simulink model "hcu_main_ADASwEPS"  (Simulink 8.2)
settings: Solver=FixedStepDiscrete  StartTime=0.0  StopTime=inf  FixedStep=0.001  RelTol=1e-3
PostLoadFcn:
  | , if any(exist('dsrtsu_mdlpostloadfcn', 'file') == [2, 3, 6]), try dsrtsu_mdlpostloadfcn('Execute', bdroot); catch fprintf('Error in PostLoadFcn (dsrtsu_mdlpostloadfcn) for model "%s":\n %s\n', bdroot, lasterr); end, end,
values from neighbouring files (symbols this model uses):
  C_TASK_1MS_S = (	C_TICK_TIME_S       )    [hcu_local_hdr.m]    (also in temp_ovrd_values.m = double(	0.001                  ))
  C_TASK_5MS_S = (	C_TICK_TIME_S      	)    [hcu_local_hdr.m]
  ENUM_ADASLFCSTATUS_OFF = uint8(  0  )    [hcu_local_hdr.m]
  ENUM_ADASLFCSTATUS_STANDBY = uint8(  1  )    [hcu_local_hdr.m]
  ENUM_ADASLKASTATUS_ACTIVE = uint8(  2  )    [hcu_local_hdr.m]
  ENUM_ADASLKASTATUS_OFF = uint8(  0  )    [hcu_local_hdr.m]
  ENUM_ADASLKASTATUS_STANDBY = uint8(  1  )    [hcu_local_hdr.m]
  ENUM_EPSMODEREQ_ANGLE = uint8(  1  )    [hcu_local_hdr.m]
  ENUM_EPSMODEREQ_INTERNAL = uint8(  0  )    [hcu_local_hdr.m]
  ENUM_EPSMODEREQ_TORQUE = uint8(  2  )    [hcu_local_hdr.m]
  ENUM_GEARPOSN_1ST = uint8(  1  )    [hcu_local_hdr.m]
  ENUM_GEARPOSN_2ND = uint8(  2  )    [hcu_local_hdr.m]
  ENUM_GEARPOSN_3RD = uint8(  3  )    [hcu_local_hdr.m]
  ENUM_GEARPOSN_4TH = uint8(  4  )    [hcu_local_hdr.m]
  ENUM_GEARPOSN_5TH = uint8(  5  )    [hcu_local_hdr.m]
  ENUM_GEARPOSN_6TH = uint8(  6  )    [hcu_local_hdr.m]
  ENUM_GEARPOSN_PN = uint8(  0  )    [hcu_local_hdr.m]
  ENUM_GEARPOSN_R = uint8(  7  )    [hcu_local_hdr.m]
  FALSE = boolean( 0 )    [hcu_local_hdr.m]
  TRUE = boolean( 1 )    [hcu_local_hdr.m]
undefined symbols (not defined in the file or in its folder): AACC_DistCtrlIMult_X_mps2, AACC_DistCtrlPMult_X_mps2, AACC_GearActual_enum, AACC_SpdCtrlIMult_X_mps2, AACC_SpdCtrlPMult_X_mps2, AACC_VehSpd_kph, AISP_EPSCurrent_pct, AISP_TqASensorDelta_pct, AISP_TqBSensorDelta_pct, ENUM_ACCSTATUS_ACTIVE, ENUM_ACCSTATUS_OFF, ENUM_ACCSTATUS_STANDBY, ENUM_ADASLFCSTATUS_ACTIVE, ENUM_ADASLFCSTATUS_TRANSITION, ENUM_LFCCCONTSTATUS_ACTIVE, ENUM_LFCCCONTSTATUS_NOTAVAIL_TEMP, ENUM_LFCCCONTSTATUS_OFF, ENUM_LFCCCONTSTATUS_READY, ENUM_LFCCCONTSTATUS_TRANSITION, ENUM_LKACCONTSTATUS_ACTIVE, ENUM_LKACCONTSTATUS_NOTAVAIL_TEMP, ENUM_LKACCONTSTATUS_OFF, ENUM_LKACCONTSTATUS_READY, KACC_AcclReqMax_g, KACC_AcclReqMin_g, KACC_ACCSetTimeGapDef1_s, KACC_ACCSetTimeGapDef2_s, KACC_ACCSetTimeGapDef3_s, KACC_ACCSetTimeGapDef4_s, KACC_ACCSetTimeGapDef5_s, KACC_AirDensity_kgpm3, KACC_AirDragCoef_rat, KACC_CommandsOn_flg, KACC_CruzSpdChgTimeThres_s, KACC_DecReqSwOffThres_Nm, KACC_DecReqSwOnThres_Nm, KACC_DistCtrlAdjTime_s, KACC_DistCtrlCalRate_s, KACC_DistCtrlIC_mps2, KACC_DistCtrlIGain_rat, KACC_DistCtrlIMax_mps2, KACC_DistCtrlIMin_mps2, KACC_DistCtrlIRest_flg, KACC_DistCtrlKGain_rat, KACC_DistCtrlPause_flg, KACC_DistCtrlPGain_rat, KACC_FinalDriveEff_pct, KACC_FinalDriveRatio_rat, KACC_FrontalArea_m2, KACC_GearBoxEff_pct, KACC_LongPushSpdChg_kph, KACC_MaxAccSetSpd_kph, KACC_MinAccSetSpd_kph, KACC_SetAllowSpdLim_kph, KACC_SpdCtrlAdjTime_s, KACC_SpdCtrlCalRate_s, KACC_SpdCtrlIC_mps2, KACC_SpdCtrlIGain_rat, KACC_SpdCtrlIMax_mps2, KACC_SpdCtrlIMin_mps2 ... (+26)
libraries: simulink x54, adas_lib x6, rti1401lib_dio_type3 x4, rtimmsu_dsrtlib x3, hcu_lib x2, aeb x1, ddm x1, dfr x1, dgi x1, dhp x1, dinr x1, dip x1
(part 9 of 9)

== system hcu_main_ADASwEPS/APPH/ACC/ACC/ACCStrategy/Torque Estimation/TqConverter ==
  TqIn_TC : Inport
  OmegaIn_TC : Inport  Port=2
  VDINR_EngSpd_rpm : Inport  Port=3
  Gain : Gain  Gain=2*pi/60
  Product1 : Product  Inputs=**  RndMeth=Zero
  Product3 : Product  Inputs=*/  RndMeth=Zero
  TorqueRatio : Lookup  InputValues=[0 0.1 0.202 0.301 0.402 0.503 0.621 0.654 0.702 0.751 0.8 0.821 0.842 0.861 0.882 0.901 0.921]  Table=|  LookUpMeth=Interpolation-Use End Values
      | [1.88 1.81 1.73 1.64 1.53 1.41 1.28 1.25 1.2 1.15 1.1 1.08 1.06 1.04 1.01 1 1
      | ]
  VACC_TqReqRaw_Nm : Outport
  wires:
  Product1/1 -> VACC_TqReqRaw_Nm/1  "VACC_TqReqRaw_Nm"
  VDINR_EngSpd_rpm/1 -> Gain/1
  OmegaIn_TC/1 -> Product3/1
  Product3/1 -> TorqueRatio/1
  TorqueRatio/1 -> Product1/2
  TqIn_TC/1 -> Product1/1
  Gain/1 -> Product3/2

== system hcu_main_ADASwEPS/APPH/ACC/ACC/ACCStrategy/Trigger signal generator/trigger signal generator ==
  Time_dur [s] : Inport
  Constant3 : Constant  Value=0  OutDataTypeStr=single
  Constant4 : Constant  Value=C_TASK_5MS_S
  Relational Operator1 : RelationalOperator  OutDataTypeStr=boolean
  Sum1 : Sum  Inputs=|++  SaturateOnIntegerOverflow=on  InputSameDT=on
  Sum2 : Sum  Inputs=+-
  Switch3 : Switch  Threshold=0.5
  Unit Delay2 : UnitDelay  SampleTime=-1
  Unit Delay3 : UnitDelay  SampleTime=-1
  Trigger_signal : Outport  OutputWhenDisabled=reset  InitialOutput=[0]
  wires:
  Sum2/1 -> Relational Operator1/2
  Unit Delay3/1 -> Switch3/2
  Unit Delay2/1 -> Sum1/2
  Switch3/1 -> Relational Operator1/1, Unit Delay2/1
  Constant3/1 -> Switch3/1
  Time_dur [s]/1 -> Sum2/1
  Relational Operator1/1 -> Unit Delay3/1, Trigger_signal/1
  Constant4/1 -> Sum2/2, Sum1/1
  Sum1/1 -> Switch3/3

== system hcu_main_ADASwEPS/APPH/ACC/ACC/ACCStrategy/Vehicle Acceleration Calculation/signal_filter ==
  raw_input : Inport
  Tc : Inport  Port=2
  Ts : Inport  Port=3
  FirstOrderFilter : Subsystem  RTWFileName=HCU_LIB
      settings: RTWFileNameOpts=User specified
  IC : UnitDelay  Tag=struct('comment',struct('text','','placement',1),'logdata',struct('maxnumvals',inf,'plotchannels',[],'stepsize',0,'downsampling',1,'loggingmode',3,'channels',1),'output',struct('width',1,'name','$S_$B','unit','','type','Int16','offset',0,'max',NaN,'min',NaN,'freeze',1,'lsb',1,'arb',0,'class','default','address','','description','','autoscalingmode',1,'lowerheadroom',1,'upperheadroom',1,'headroomunit','bit','checkmin',0,'checkmax',0,'show',0,'initial','2'),'state',0,'dt','-1','date',731455.586925799)  SampleTime=-1
  Switch1 : Switch  Tag=struct('comment',struct('text','','placement',1),'logdata',struct('maxnumvals',inf,'plotchannels',[],'stepsize',0,'downsampling',1,'loggingmode',3,'channels',1),'output',struct('width',1,'name','$S_$B','unit','','type','Int32Bin15','offset',0,'max',65535,'min',-65536,'freeze',1,'lsb',2^-15,'arb',0,'class','default','address','','description','','autoscalingmode',1,'lowerheadroom',1,'upperheadroom',1,'headroomunit','bit','checkmin',0,'checkmax',0,'show',0),'threshold',struct('width',1,'name','$S_$B_threshold','unit','','type','Int16','offset',0,'max',NaN,'min',NaN,'freeze',1,'lsb',1,'arb',0,'class','default','address','','description','','value','1','scalar',0),'date',731455.58657044)  Threshold=0.5  InputSameDT=on
  zero : Constant  Tag=struct('comment',struct('text','','placement',1),'output',struct('width',1,'name','$S_$B','unit','','type','Int16','offset',0,'max',NaN,'min',NaN,'freeze',1,'lsb',1,'arb',0,'class','default','address','','description','','value','0','tolerance',1,'show',0),'date',731455.58675544)  Value=TRUE
  zero1 : Constant  Tag=struct('comment',struct('text','','placement',1),'output',struct('width',1,'name','$S_$B','unit','','type','Int16','offset',0,'max',NaN,'min',NaN,'freeze',1,'lsb',1,'arb',0,'class','default','address','','description','','value','0','tolerance',1,'show',0),'date',731455.58675544)  Value=0  OutDataTypeStr=single
  raw_input_filt : Outport
  wires:
  zero/1 -> IC/1
  raw_input/1 -> FirstOrderFilter/1(in)
  Tc/1 -> Switch1/1
  Ts/1 -> FirstOrderFilter/3(Ts)
  IC/1 -> Switch1/2
  FirstOrderFilter/1(out) -> raw_input_filt/1
  Switch1/1 -> FirstOrderFilter/2(Tc)
  zero1/1 -> Switch1/3

== system hcu_main_ADASwEPS/EPSS/EPSS/AngleMode/Angle2Torque/Rate_Limit/RateLimiter ==
  Data_Input : Inport
  Rising Rate : Inport  Port=2
  Falling Rate : Inport  Port=3
  Initial_Condition : Inport  Port=4
  Chart : Stateflow chart  TreatAsAtomicUnit=on
  Constant : Constant  Value=C_TASK_1MS_S
  Constant1 : Constant  Value=C_TASK_1MS_S
  Constant4 : Constant
  Constant5 : Constant
  Data Type Conversion : DataTypeConversion  OutDataTypeStr=boolean
  Data Type Conversion1 : DataTypeConversion  OutDataTypeStr=boolean
  Product{1..4} (4 alike) : Product  Inputs=*/  RndMeth=Zero
  Relational Operator : RelationalOperator  Operator=>  OutDataTypeStr=boolean
  Relational Operator1 : RelationalOperator  Operator=<  OutDataTypeStr=boolean
  Saturation : Subsystem
  Sum1 : Sum  Inputs=|++
  Switch1 : Switch  Threshold=0.5
  Unit Delay1 : UnitDelay  SampleTime=-1
  Data_Output : Outport
  wires:
  Relational Operator1/1 -> Data Type Conversion/1
  Relational Operator/1 -> Data Type Conversion1/1
  Data_Input/1 -> Relational Operator/1, Relational Operator1/1, Chart/3(Data_in)
  Product3/1 -> Product1/2
  Product4/1 -> Product2/2
  Product1/1 -> Chart/4(increase_tou)
  Product2/1 -> Chart/5(decrease_tou)
  Data Type Conversion/1 -> Chart/2(decrease)
  Data Type Conversion1/1 -> Chart/1(increase)
  Chart/2(tou) -> Sum1/1
  Saturation/1(out) -> Switch1/3
  Chart/3(Min) -> Saturation/2(min)
  Chart/4(Max) -> Saturation/3(max)
  Chart/1(Initial) -> Switch1/2
  Initial_Condition/1 -> Switch1/1
  Constant/1 -> Product3/2
  Constant4/1 -> Product3/1
  Constant1/1 -> Product4/2
  Constant5/1 -> Product4/1
  Switch1/1 -> Data_Output/1, Unit Delay1/1
  Rising Rate/1 -> Product1/1
  Falling Rate/1 -> Product2/1
  Sum1/1 -> Saturation/1(in)
  Unit Delay1/1 -> Sum1/2, Relational Operator/2, Relational Operator1/2

== system hcu_main_ADASwEPS/APPH/ACC/ACC/ACCStrategy/Distance Control/PI Controller for Distance Control/Integrator ==
  In : Inport
  Rst : Inport  Port=2
  IC : Inport  Port=3
  Min : Inport  Port=4
  Max : Inport  Port=5
  Constant : Constant  Value=C_TASK_5MS_S  OutDataTypeStr=single
  Data Type Conversion : DataTypeConversion  OutDataTypeStr=boolean  RndMeth=Zero
  Product : Product  SaturateOnIntegerOverflow=on  InputSameDT=on  OutDataTypeStr=Inherit: Same as first input
  Saturation : Subsystem
  Sum : Sum  Inputs=++|  SaturateOnIntegerOverflow=on  InputSameDT=on
  Switch1 : Switch  Threshold=1  ZeroCross=off  SaturateOnIntegerOverflow=on  InputSameDT=on
  Unit Delay : UnitDelay  SampleTime=-1
  Out : Outport
  wires:
  IC/1 -> Switch1/1
  Max/1 -> Saturation/3(max)
  Min/1 -> Saturation/2(min)
  Data Type Conversion/1 -> Switch1/2
  Rst/1 -> Data Type Conversion/1
  Unit Delay/1 -> Switch1/3
  Product/1 -> Sum/2
  In/1 -> Product/1
  Constant/1 -> Product/2
  Switch1/1 -> Sum/1, Out/1
  Sum/1 -> Saturation/1(in)
  Saturation/1(out) -> Unit Delay/1

== system hcu_main_ADASwEPS/APPH/ACC/ACC/ACCStrategy/Distance Control/Trigger signal generator/trigger signal generator ==
  Time_dur [s] : Inport
  Constant3 : Constant  Value=0  OutDataTypeStr=single
  Constant4 : Constant  Value=C_TASK_5MS_S
  Relational Operator1 : RelationalOperator  OutDataTypeStr=boolean
  Sum1 : Sum  Inputs=|++  SaturateOnIntegerOverflow=on  InputSameDT=on
  Sum2 : Sum  Inputs=+-
  Switch3 : Switch  Threshold=0.5
  Unit Delay2 : UnitDelay  SampleTime=-1
  Unit Delay3 : UnitDelay  SampleTime=-1
  Trigger_signal : Outport  OutputWhenDisabled=reset  InitialOutput=[0]
  wires:
  Sum2/1 -> Relational Operator1/2
  Unit Delay3/1 -> Switch3/2
  Unit Delay2/1 -> Sum1/2
  Switch3/1 -> Relational Operator1/1, Unit Delay2/1
  Constant3/1 -> Switch3/1
  Time_dur [s]/1 -> Sum2/1
  Relational Operator1/1 -> Unit Delay3/1, Trigger_signal/1
  Constant4/1 -> Sum2/2, Sum1/1
  Sum1/1 -> Switch3/3

== system hcu_main_ADASwEPS/APPH/ACC/ACC/ACCStrategy/Distance Control/Trigger signal generator1/trigger signal generator ==
  Time_dur [s] : Inport
  Constant3 : Constant  Value=0  OutDataTypeStr=single
  Constant4 : Constant  Value=C_TASK_5MS_S
  Relational Operator1 : RelationalOperator  OutDataTypeStr=boolean
  Sum1 : Sum  Inputs=|++  SaturateOnIntegerOverflow=on  InputSameDT=on
  Sum2 : Sum  Inputs=+-
  Switch3 : Switch  Threshold=0.5
  Unit Delay2 : UnitDelay  SampleTime=-1
  Unit Delay3 : UnitDelay  SampleTime=-1
  Trigger_signal : Outport  OutputWhenDisabled=reset  InitialOutput=[0]
  wires:
  Sum2/1 -> Relational Operator1/2
  Unit Delay3/1 -> Switch3/2
  Unit Delay2/1 -> Sum1/2
  Switch3/1 -> Relational Operator1/1, Unit Delay2/1
  Constant3/1 -> Switch3/1
  Time_dur [s]/1 -> Sum2/1
  Relational Operator1/1 -> Unit Delay3/1, Trigger_signal/1
  Constant4/1 -> Sum2/2, Sum1/1
  Sum1/1 -> Switch3/3

== system hcu_main_ADASwEPS/APPH/ACC/ACC/ACCStrategy/Distance Control/Vehicle Acceleration Calculation/signal_filter ==
  raw_input : Inport
  Tc : Inport  Port=2
  Ts : Inport  Port=3
  FirstOrderFilter : Subsystem  RTWFileName=HCU_LIB
      settings: RTWFileNameOpts=User specified
  IC : UnitDelay  Tag=struct('comment',struct('text','','placement',1),'logdata',struct('maxnumvals',inf,'plotchannels',[],'stepsize',0,'downsampling',1,'loggingmode',3,'channels',1),'output',struct('width',1,'name','$S_$B','unit','','type','Int16','offset',0,'max',NaN,'min',NaN,'freeze',1,'lsb',1,'arb',0,'class','default','address','','description','','autoscalingmode',1,'lowerheadroom',1,'upperheadroom',1,'headroomunit','bit','checkmin',0,'checkmax',0,'show',0,'initial','2'),'state',0,'dt','-1','date',731455.586925799)  SampleTime=-1
  Switch1 : Switch  Tag=struct('comment',struct('text','','placement',1),'logdata',struct('maxnumvals',inf,'plotchannels',[],'stepsize',0,'downsampling',1,'loggingmode',3,'channels',1),'output',struct('width',1,'name','$S_$B','unit','','type','Int32Bin15','offset',0,'max',65535,'min',-65536,'freeze',1,'lsb',2^-15,'arb',0,'class','default','address','','description','','autoscalingmode',1,'lowerheadroom',1,'upperheadroom',1,'headroomunit','bit','checkmin',0,'checkmax',0,'show',0),'threshold',struct('width',1,'name','$S_$B_threshold','unit','','type','Int16','offset',0,'max',NaN,'min',NaN,'freeze',1,'lsb',1,'arb',0,'class','default','address','','description','','value','1','scalar',0),'date',731455.58657044)  Threshold=0.5  InputSameDT=on
  zero : Constant  Tag=struct('comment',struct('text','','placement',1),'output',struct('width',1,'name','$S_$B','unit','','type','Int16','offset',0,'max',NaN,'min',NaN,'freeze',1,'lsb',1,'arb',0,'class','default','address','','description','','value','0','tolerance',1,'show',0),'date',731455.58675544)  Value=TRUE
  zero1 : Constant  Tag=struct('comment',struct('text','','placement',1),'output',struct('width',1,'name','$S_$B','unit','','type','Int16','offset',0,'max',NaN,'min',NaN,'freeze',1,'lsb',1,'arb',0,'class','default','address','','description','','value','0','tolerance',1,'show',0),'date',731455.58675544)  Value=0  OutDataTypeStr=single
  raw_input_filt : Outport
  wires:
  zero/1 -> IC/1
  raw_input/1 -> FirstOrderFilter/1(in)
  Tc/1 -> Switch1/1
  Ts/1 -> FirstOrderFilter/3(Ts)
  IC/1 -> Switch1/2
  FirstOrderFilter/1(out) -> raw_input_filt/1
  Switch1/1 -> FirstOrderFilter/2(Tc)
  zero1/1 -> Switch1/3

== system hcu_main_ADASwEPS/APPH/ACC/ACC/ACCStrategy/Speed Control/PI Controller for Seepd Control/Integrator ==
  In : Inport
  Rst : Inport  Port=2
  IC : Inport  Port=3
  Min : Inport  Port=4
  Max : Inport  Port=5
  Constant : Constant  Value=C_TASK_5MS_S  OutDataTypeStr=single
  Data Type Conversion : DataTypeConversion  OutDataTypeStr=boolean  RndMeth=Zero
  Product : Product  SaturateOnIntegerOverflow=on  InputSameDT=on  OutDataTypeStr=Inherit: Same as first input
  Saturation : Subsystem
  Sum : Sum  Inputs=++|  SaturateOnIntegerOverflow=on  InputSameDT=on
  Switch1 : Switch  Threshold=1  ZeroCross=off  SaturateOnIntegerOverflow=on  InputSameDT=on
  Unit Delay : UnitDelay  SampleTime=-1
  Out : Outport
  wires:
  IC/1 -> Switch1/1
  Max/1 -> Saturation/3(max)
  Min/1 -> Saturation/2(min)
  Data Type Conversion/1 -> Switch1/2
  Rst/1 -> Data Type Conversion/1
  Unit Delay/1 -> Switch1/3
  Product/1 -> Sum/2
  In/1 -> Product/1
  Constant/1 -> Product/2
  Switch1/1 -> Sum/1, Out/1
  Sum/1 -> Saturation/1(in)
  Saturation/1(out) -> Unit Delay/1

== system hcu_main_ADASwEPS/APPH/ACC/ACC/ACCStrategy/Speed Control/Trigger signal generator/trigger signal generator ==
  Time_dur [s] : Inport
  Constant3 : Constant  Value=0  OutDataTypeStr=single
  Constant4 : Constant  Value=C_TASK_5MS_S
  Relational Operator1 : RelationalOperator  OutDataTypeStr=boolean
  Sum1 : Sum  Inputs=|++  SaturateOnIntegerOverflow=on  InputSameDT=on
  Sum2 : Sum  Inputs=+-
  Switch3 : Switch  Threshold=0.5
  Unit Delay2 : UnitDelay  SampleTime=-1
  Unit Delay3 : UnitDelay  SampleTime=-1
  Trigger_signal : Outport  OutputWhenDisabled=reset  InitialOutput=[0]
  wires:
  Sum2/1 -> Relational Operator1/2
  Unit Delay3/1 -> Switch3/2
  Unit Delay2/1 -> Sum1/2
  Switch3/1 -> Relational Operator1/1, Unit Delay2/1
  Constant3/1 -> Switch3/1
  Time_dur [s]/1 -> Sum2/1
  Relational Operator1/1 -> Unit Delay3/1, Trigger_signal/1
  Constant4/1 -> Sum2/2, Sum1/1
  Sum1/1 -> Switch3/3

== system hcu_main_ADASwEPS/APPH/ACC/ACC/ACCStrategy/Torque Estimation/Tire/Derivative ==
  SampleTime : Inport
  Omega_tire : Inport  Port=2
  Trigger : TriggerPort
  Divide : Product  Inputs=*/
  Mux1 : Mux  Inputs=2
  Scope1 : Scope
      settings: SaveName=ScopeData9
  Subtract : Sum  Inputs=+-
  Unit Delay : UnitDelay  SampleTime=-1
  AlphaOut_tire : Outport
  wires:
  Omega_tire/1 -> Subtract/1, Unit Delay/1
  Divide/1 -> AlphaOut_tire/1
  SampleTime/1 -> Divide/2
  Subtract/1 -> Divide/1, Mux1/1
  Unit Delay/1 -> Subtract/2, Mux1/2
  Mux1/1 -> Scope1/1

== system hcu_main_ADASwEPS/APPH/ACC/ACC/ACCStrategy/Torque Estimation/Tire/trigger signal generator ==
  Time_dur [s] : Inport
  Constant3 : Constant  Value=single(0)
  Constant4 : Constant  Value=C_TASK_5MS_S
  Relational Operator1 : RelationalOperator  OutDataTypeStr=boolean
  Sum1 : Sum  Inputs=|++  SaturateOnIntegerOverflow=on  InputSameDT=on
  Sum2 : Sum  Inputs=+-
  Switch3 : Switch  Threshold=0.5
  Unit Delay2 : UnitDelay  InitialCondition=single(0)  SampleTime=-1
  Unit Delay3 : UnitDelay  SampleTime=-1
  Trigger_signal : Outport  OutputWhenDisabled=reset  InitialOutput=[0]
  wires:
  Sum1/1 -> Switch3/3
  Constant4/1 -> Sum1/1, Sum2/2
  Relational Operator1/1 -> Trigger_signal/1, Unit Delay3/1
  Time_dur [s]/1 -> Sum2/1
  Constant3/1 -> Switch3/1
  Switch3/1 -> Unit Delay2/1, Relational Operator1/1
  Unit Delay2/1 -> Sum1/2
  Unit Delay3/1 -> Switch3/2
  Sum2/1 -> Relational Operator1/2

== system hcu_main_ADASwEPS/APPH/ACC/ACC/ACCStrategy/Vehicle Acceleration Calculation/signal_filter/FirstOrderFilter ==
  in : Inport
  Tc : Inport  Port=2
  Ts : Inport  Port=3
  Add : Sum
  Add1 : Sum
  Add2 : Sum  Inputs=+-
  Constant : Constant  OutDataTypeStr=single
  Divide : Product  Inputs=*/
  Product : Product  RndMeth=Zero
  Product1 : Product  RndMeth=Zero
  Unit Delay : UnitDelay  SampleTime=-1
  out : Outport
  wires:
  Add/1 -> Unit Delay/1, out/1
  Product1/1 -> Add/2
  Product/1 -> Add/1
  Add2/1 -> Product/2
  in/1 -> Product/1
  Divide/1 -> Product1/1, Add2/2
  Constant/1 -> Add2/1
  Add1/1 -> Divide/2
  Ts/1 -> Add1/2
  Tc/1 -> Divide/1, Add1/1
  Unit Delay/1 -> Product1/2

== system hcu_main_ADASwEPS/EPSS/EPSS/AngleMode/Angle2Torque/Rate_Limit/RateLimiter/Saturation ==
  in : Inport
  min : Inport  Port=2
  max : Inport  Port=3
  MinMax : MinMax  Function=max  Inputs=2  ZeroCross=off  SaturateOnIntegerOverflow=on  InputSameDT=on
  MinMax1 : MinMax  Inputs=2  ZeroCross=off  SaturateOnIntegerOverflow=on  InputSameDT=on
  out : Outport
  wires:
  MinMax1/1 -> out/1
  max/1 -> MinMax1/2
  min/1 -> MinMax/2
  in/1 -> MinMax/1
  MinMax/1 -> MinMax1/1

== system hcu_main_ADASwEPS/APPH/ACC/ACC/ACCStrategy/Distance Control/PI Controller for Distance Control/Integrator/Saturation ==
  in : Inport
  min : Inport  Port=2
  max : Inport  Port=3
  MinMax : MinMax  Function=max  Inputs=2  ZeroCross=off  SaturateOnIntegerOverflow=on  InputSameDT=on
  MinMax1 : MinMax  Inputs=2  ZeroCross=off  SaturateOnIntegerOverflow=on  InputSameDT=on
  out : Outport
  wires:
  MinMax/1 -> MinMax1/1
  in/1 -> MinMax/1
  min/1 -> MinMax/2
  max/1 -> MinMax1/2
  MinMax1/1 -> out/1

== system hcu_main_ADASwEPS/APPH/ACC/ACC/ACCStrategy/Distance Control/Vehicle Acceleration Calculation/signal_filter/FirstOrderFilter ==
  in : Inport
  Tc : Inport  Port=2
  Ts : Inport  Port=3
  Add : Sum
  Add1 : Sum
  Add2 : Sum  Inputs=+-
  Constant : Constant  OutDataTypeStr=single
  Divide : Product  Inputs=*/
  Product : Product  RndMeth=Zero
  Product1 : Product  RndMeth=Zero
  Unit Delay : UnitDelay  SampleTime=-1
  out : Outport
  wires:
  Add/1 -> Unit Delay/1, out/1
  Product1/1 -> Add/2
  Product/1 -> Add/1
  Add2/1 -> Product/2
  in/1 -> Product/1
  Divide/1 -> Product1/1, Add2/2
  Constant/1 -> Add2/1
  Add1/1 -> Divide/2
  Ts/1 -> Add1/2
  Tc/1 -> Divide/1, Add1/1
  Unit Delay/1 -> Product1/2

== system hcu_main_ADASwEPS/APPH/ACC/ACC/ACCStrategy/Speed Control/PI Controller for Seepd Control/Integrator/Saturation ==
  in : Inport
  min : Inport  Port=2
  max : Inport  Port=3
  MinMax : MinMax  Function=max  Inputs=2  ZeroCross=off  SaturateOnIntegerOverflow=on  InputSameDT=on
  MinMax1 : MinMax  Inputs=2  ZeroCross=off  SaturateOnIntegerOverflow=on  InputSameDT=on
  out : Outport
  wires:
  MinMax/1 -> MinMax1/1
  in/1 -> MinMax/1
  min/1 -> MinMax/2
  max/1 -> MinMax1/2
  MinMax1/1 -> out/1

== stateflow chart APPH/Scheduler ==
  (default) -> (junction 23)
  (junction 23) -> (junction 24) : {
      | trig_PMM; ...
      | trig_DGI; ...
      | trig_DINR; ...
      | trig_TRCK; ...
      | trig_DDM; ...
      | trig_DHP; ...
      | trig_EID; ...
      | trig_LANE; ...
      | trig_SFTY; ...
      | trig_FST; ...
      | trig_LFCM; ...
      | trig_STR; ...
      | trig_OBJ; ...
      | trig_PTH; ...
      | trig_MCT;...
      | trig_TTC; ...
      | trig_AEB; ...
      | trig_ACC; ...
      | trig_DIP; ...
      | trig_DFR; ...
      | }
  events: trig_PMM output FUNCTION_CALL_EVENT; trig_DGI output FUNCTION_CALL_EVENT; trig_DINR output FUNCTION_CALL_EVENT; trig_TRCK output FUNCTION_CALL_EVENT; trig_DDM output FUNCTION_CALL_EVENT; trig_DHP output FUNCTION_CALL_EVENT; trig_EID output FUNCTION_CALL_EVENT; trig_LANE output FUNCTION_CALL_EVENT; trig_SFTY output FUNCTION_CALL_EVENT; trig_FST output FUNCTION_CALL_EVENT; trig_LFCM output FUNCTION_CALL_EVENT; trig_STR output FUNCTION_CALL_EVENT; trig_OBJ output FUNCTION_CALL_EVENT; trig_PTH output FUNCTION_CALL_EVENT; trig_MCT output FUNCTION_CALL_EVENT; trig_TTC output FUNCTION_CALL_EVENT; trig_AEB output FUNCTION_CALL_EVENT; trig_ACC output FUNCTION_CALL_EVENT; trig_DIP output FUNCTION_CALL_EVENT; trig_DFR output FUNCTION_CALL_EVENT

== stateflow chart APPH/ACC/ACC/ACCStatus_SetSpeed_SetTimeGap/ACC_SetSpeed_Determination ==
  state ACCOff
    en:VACC_ACCSetSpd_kph=0;
    en:VACC_ACCSetSpdIni_kph=0;
    en:CurrSetSpd=0;
  state Initialize
    en:VACC_ACCSetSpd_kph=0;
    en:VACC_ACCSetSpdIni_kph=0;
    en:CurrSetSpd=0;
  state ACCOn
    state SetOn
      en:VACC_ACCSetSpd_kph=VDINR_VehSpd_kph;
      en:VACC_ACCSetSpdIni_kph=VDINR_VehSpd_kph;
      en:CurrSetSpd=VDINR_VehSpd_kph;
    state SetOn_HighSpeed
      en:VACC_ACCSetSpd_kph=VACC_MaxAccSetSpd_kph;
      en:VACC_ACCSetSpdIni_kph=VACC_MaxAccSetSpd_kph;
      en:CurrSetSpd=VACC_MaxAccSetSpd_kph;
    state SetOn_LowSpeed
      en:VACC_ACCSetSpd_kph=VACC_MinAccSetSpd_kph;
      en:VACC_ACCSetSpdIni_kph=VACC_MinAccSetSpd_kph;
      en:CurrSetSpd=VACC_MinAccSetSpd_kph;
    state ResOn
      en:VACC_ACCSetSpd_kph=VACC_ACCSetSpdLast_kph;
      en:VACC_ACCSetSpdIni_kph=VACC_ACCSetSpdLast_kph;
      en:CurrSetSpd=VACC_ACCSetSpdLast_kph;
    state WaitforACCActive
      en:VACC_ACCSetSpd_kph=CurrSetSpd;
      en:VACC_ACCSetSpdIni_kph=CurrSetSpd;
    state BrakeSet_LowSpeed
      en:VACC_ACCSetSpd_kph=VACC_MinAccSetSpd_kph;
      en:VACC_ACCSetSpdIni_kph=VACC_MinAccSetSpd_kph;
      en:CurrSetSpd=VACC_MinAccSetSpd_kph;
    state BrakeSet_NormalSpeed
      en:VACC_ACCSetSpd_kph=CurrSetSpd;
      en:VACC_ACCSetSpdIni_kph=CurrSetSpd;
    state SpeedSet
      state WaitingForSpdChange
        en:VACC_ACCSetSpd_kph=CurrSetSpd;
        en:VACC_ACCSetSpdIni_kph=CurrSetSpd;
      state PrepareToDec
      state PrepareToInc
      state DecreaseToMin
        en: CurrSetSpd=VACC_MinAccSetSpd_kph;
        en: VACC_ACCSetSpd_kph=CurrSetSpd;
      state Decrease1
        ex: CurrSetSpd=CurrSetSpd-1;
      state Decrease11
        en: CurrSetSpd=CurrSetSpd-VACC_LongPushSpdChg_kph;
        en: VACC_ACCSetSpd_kph=CurrSetSpd;
      state Increase1
        ex: CurrSetSpd=CurrSetSpd+1;
      state SetSpeedUpLimit
        ex: CurrSetSpd=VOBU_SetSpdUplim_kph;
      (default) -> WaitingForSpdChange
      SetSpeedUpLimit -> WaitingForSpdChange
      Increase1 -> WaitingForSpdChange
      (junction 89) -> WaitingForSpdChange [order 2]
      WaitingForSpdChange -> PrepareToInc [order 2] : [VACC_ACCResSpdIncVCU_flg]
      (junction 90) -> WaitingForSpdChange [order 2]
      DecreaseToMin -> WaitingForSpdChange : [!VACC_ACCSetSpdDecVCU_flg]
      Decrease11 -> WaitingForSpdChange [order 2] : [!VACC_ACCSetSpdDecVCU_flg]
      WaitingForSpdChange -> PrepareToDec [order 1] : [VACC_ACCSetSpdDecVCU_flg]
      (junction 88) -> WaitingForSpdChange [order 2]
      Decrease1 -> WaitingForSpdChange
      PrepareToDec -> (junction 86) [order 2] : after(VACC_CruzSpdChgTimeThres_s/C_TASK_5MS_S,tick) ...
          | [VACC_ACCSetSpdDecVCU_flg]
      (junction 86) -> (junction 87) [order 1] : [CurrSetSpd>=(VACC_MinAccSetSpd_kph+1) && ...
          |  CurrSetSpd<(VACC_MinAccSetSpd_kph+VACC_LongPushSpdChg_kph)]
      PrepareToInc -> (junction 90) [order 1] : after(VACC_CruzSpdChgTimeThres_s/C_TASK_5MS_S,tick)...
          | [!VACC_ACCResSpdIncVCU_flg]
      (junction 86) -> Decrease11 [order 2] : [CurrSetSpd>=(VACC_MinAccSetSpd_kph+VACC_LongPushSpdChg_kph)]
      (junction 87) -> DecreaseToMin
      PrepareToDec -> (junction 88) [order 1] : [!VACC_ACCSetSpdDecVCU_flg]
      PrepareToInc -> (junction 89) [order 2] : [!VACC_ACCResSpdIncVCU_flg]
      (junction 88) -> Decrease1 [order 1] : [CurrSetSpd>=(VACC_MinAccSetSpd_kph+1)]
      (junction 89) -> Increase1 [order 1] : [CurrSetSpd<=(VACC_MaxAccSetSpd_kph-1)]
      (junction 93) -> Decrease11
      (junction 90) -> (junction 94) [order 1] : [CurrSetSpd<=(VOBU_SetSpdUplim_kph)]
      Decrease11 -> (junction 92) [order 1] : after(VACC_CruzSpdChgTimeThres_s/C_TASK_5MS_S,tick) ...
          | [VACC_ACCSetSpdDecVCU_flg]
      (junction 91) -> DecreaseToMin
      (junction 92) -> (junction 91) [order 1] : [CurrSetSpd>=(VACC_MinAccSetSpd_kph+1) && ...
          |  CurrSetSpd<(VACC_MinAccSetSpd_kph+VACC_LongPushSpdChg_kph)]
      (junction 92) -> (junction 93) [order 2] : [CurrSetSpd>=(VACC_MinAccSetSpd_kph+VACC_LongPushSpdChg_kph)]
      (junction 94) -> SetSpeedUpLimit
    (default) -> WaitforACCActive
    (junction 48) -> WaitforACCActive
    (junction 59) -> (junction 48)
    WaitforACCActive -> (junction 49)
    (junction 49) -> (junction 50) [order 2] : [(VACC_ACCResSpdIncVCU_flg || VACC_ACCSetSpdDecVCU_flg) && VDINR_DriverBrakPedalOn_flg && VACC_InPNGear_flg && (VDINR_VehSpd_kph<VACC_SetAllowSpdLim_kph) && CurrSetSpd>=VACC_MinAccSetSpd_kph]
    (junction 49) -> (junction 51) [order 1]
    (junction 50) -> BrakeSet_NormalSpeed
    (junction 51) -> (junction 52) [order 2] : [(VACC_ACCResSpdIncVCU_flg || VACC_ACCSetSpdDecVCU_flg) && VDINR_DriverBrakPedalOn_flg && VACC_InPNGear_flg && (VDINR_VehSpd_kph<VACC_SetAllowSpdLim_kph) && CurrSetSpd<VACC_MinAccSetSpd_kph]
    (junction 51) -> (junction 53) [order 1] : [VACC_ACCActivated_flg]
    (junction 52) -> BrakeSet_LowSpeed
    (junction 53) -> (junction 54) [order 1] : [VACC_ACCResOn_flg]
    (junction 53) -> (junction 55) [order 2] : [!VACC_ACCResOn_flg]
    (junction 54) -> ResOn
    (junction 55) -> (junction 56) [order 1] : [VDINR_VehSpd_kph<VACC_MinAccSetSpd_kph]
    (junction 55) -> (junction 57) [order 2]
    (junction 56) -> SetOn_LowSpeed
    (junction 57) -> (junction 58) [order 1] : [VDINR_VehSpd_kph>VACC_MaxAccSetSpd_kph]
    (junction 57) -> SetOn [order 2]
    (junction 58) -> SetOn_HighSpeed
    SetOn -> SpeedSet : [!VACC_ACCSetSpdDecVCU_flg &&...
        | !VACC_ACCResSpdIncVCU_flg]
    SetOn_HighSpeed -> SpeedSet : [!VACC_ACCSetSpdDecVCU_flg &&...
        | !VACC_ACCResSpdIncVCU_flg]
    SetOn_LowSpeed -> SpeedSet : [!VACC_ACCSetSpdDecVCU_flg &&...
        | !VACC_ACCResSpdIncVCU_flg]
    ResOn -> SpeedSet : [!VACC_ACCSetSpdDecVCU_flg &&...
        | !VACC_ACCResSpdIncVCU_flg]
    BrakeSet_LowSpeed -> SpeedSet : [!VACC_ACCSetSpdDecVCU_flg &&...
        | !VACC_ACCResSpdIncVCU_flg]
    BrakeSet_NormalSpeed -> SpeedSet : [!VACC_ACCSetSpdDecVCU_flg &&...
        | !VACC_ACCResSpdIncVCU_flg]
    SpeedSet -> (junction 59) : [!VACC_ACCActivated_flg && ...
        | (!VDINR_DriverBrakPedalOn_flg || ...
        | VDINR_VehSpd_kph>=VACC_SetAllowSpdLim_kph || ...
        | !VACC_InPNGear_flg)]
  (default) -> Initialize
  Initialize -> ACCOn : [VACC_ACCStatus_enum==ENUM_ACCSTATUS_STANDBY || ...
      | VACC_ACCStatus_enum==ENUM_ACCSTATUS_ACTIVE]
  ACCOff -> ACCOn : [VACC_ACCStatus_enum==ENUM_ACCSTATUS_STANDBY || ...
      | VACC_ACCStatus_enum==ENUM_ACCSTATUS_ACTIVE]
  ACCOn -> ACCOff : [VACC_ACCStatus_enum==ENUM_ACCSTATUS_OFF]
  data: VACC_ACCStatus_enum input double; VACC_ACCActivated_flg input double; VACC_ACCResOn_flg input double; VDINR_DriverBrakPedalOn_flg input double; VACC_ACCSetSpd_kph output double; VDINR_VehSpd_kph input double; VACC_ACCSetSpdDecVCU_flg input double; VACC_ACCResSpdIncVCU_flg input double; VACC_InPNGear_flg input double; VACC_CruzSpdChgTimeThres_s input double; VACC_LongPushSpdChg_kph input double; VACC_MaxAccSetSpd_kph input double; VACC_MinAccSetSpd_kph input double; VOBU_SetSpdUplim_kph input double; VACC_SetAllowSpdLim_kph input double; VACC_ACCSetSpdIni_kph output single; VACC_ACCSetSpdLast_kph input double; CurrSetSpd local single; C_TASK_5MS_S parameter double; ENUM_ACCSTATUS_STANDBY parameter double; ENUM_ACCSTATUS_ACTIVE parameter double; ENUM_ACCSTATUS_OFF parameter double

== stateflow chart Scheduler ==
  settings: sampleTime=0.003125
  (default) -> (junction 168)
  (junction 168) -> (junction 169) : {
      | b1ms_count = b1ms_count +1; ...
      | b5ms_count = b5ms_count +1; ...
      | trig_LIDR; ...
      | trig_Hw_In; ...
      | trig_ISP; ...
      | trig_EPSS; ...
      | trig_OSP; ...
      | trig_Hw_Out; ...
      | }
  (junction 169) -> (junction 170) [order 1] : [b1ms_count == 2]
  (junction 169) -> (junction 171) [order 2]
  (junction 170) -> (junction 172) : /*1m_sec*/
      | {
      | b1ms_count = 0; ...
      | }
  (junction 172) -> (junction 171)
  (junction 171) -> (junction 173)
  (junction 173) -> (junction 174) [order 1] : [b5ms_count == 5]
  (junction 173) -> (junction 175) [order 2]
  (junction 174) -> (junction 176) : /*5m_sec*/
      | {
      | b5ms_count = 0; ...
      | trig_CAN; ...
      | trig_HAL; ...
      | trig_INP; ...
      | trig_APP; ...
      | trig_OUTP; ...
      | }
  (junction 176) -> (junction 175)
  (junction 175) -> (junction 177)
  (junction 177) -> (junction 178) [order 1] : [b30ms_count == 6]
  (junction 177) -> (junction 179) [order 2]
  (junction 178) -> (junction 180) : /*30m_sec*/
      | {
      | b30ms_count = 0;
      | }
  (junction 180) -> (junction 179)
  (junction 179) -> (junction 181)
  (junction 181) -> (junction 182) [order 1] : [b40ms_count == 8]
  (junction 181) -> (junction 183) [order 2]
  (junction 182) -> (junction 184) : /*40m_sec*/
      | {
      | b40ms_count = 0;
      | }
  (junction 184) -> (junction 183)
  (junction 183) -> (junction 185)
  (junction 185) -> (junction 186) [order 1] : [b100ms_count == 20]
  (junction 185) -> (junction 187) [order 2]
  (junction 186) -> (junction 188) : /*100m_sec*/
      | {
      | b100ms_count = 0;
      | }
  (junction 188) -> (junction 187)
  (junction 187) -> (junction 189)
  (junction 189) -> (junction 190) [order 1] : [b200ms_count == 40]
  (junction 189) -> (junction 191) [order 2]
  (junction 190) -> (junction 192) : /*200m_sec*/
      | {
      | b200ms_count = 0;
      | }
  (junction 192) -> (junction 191)
  data: b10ms_count local uint8; b5ms_count local uint8; b30ms_count local uint8; b40ms_count local uint8; b100ms_count local uint8; b200ms_count local uint8; b1ms_count local double
  events: trig_Hw_In output FUNCTION_CALL_EVENT; trig_ISP output FUNCTION_CALL_EVENT; trig_EPSS output FUNCTION_CALL_EVENT; trig_OSP output FUNCTION_CALL_EVENT; trig_Hw_Out output FUNCTION_CALL_EVENT; trig_LIDR output FUNCTION_CALL_EVENT; trig_HAL output FUNCTION_CALL_EVENT; trig_INP output FUNCTION_CALL_EVENT; trig_APP output FUNCTION_CALL_EVENT; trig_OUTP output FUNCTION_CALL_EVENT; trig_CAN output FUNCTION_CALL_EVENT

== stateflow chart APPH/ACC/ACC/ACCStatus_SetSpeed_SetTimeGap/ACC_SetTimeGap_Selection ==
  state Initialize
    en:VACC_ACCSetTimeGap_enum=uint8(0);
    en:VACC_ACCSetTimeGapTmp_enum=VACC_ACCSetTimeGap_enum;
    en:TimeGapPosn=uint8(4);
  state ACCOff
    en:VACC_ACCSetTimeGap_enum=uint8(0);
    en:VACC_ACCSetTimeGapTmp_enum=VACC_ACCSetTimeGap_enum;
    en:TimeGapPosn=uint8(4);
  state ACCOn
    state SetOn
      en:VACC_ACCSetTimeGap_enum=uint8(4);
      en:VACC_ACCSetTimeGapTmp_enum=VACC_ACCSetTimeGap_enum;
      en:TimeGapPosn=uint8(4);
    state ResOn
      en:VACC_ACCSetTimeGap_enum=TimeGapPosn;
      en:VACC_ACCSetTimeGapTmp_enum=VACC_ACCSetTimeGap_enum;
    state WaitforACCActive
      en:VACC_ACCSetTimeGap_enum=TimeGapPosn;
      en:VACC_ACCSetTimeGapTmp_enum=VACC_ACCSetTimeGap_enum;
      en:VACC_ACCSetTimeGapSignIni_flg=FALSE;
    state BrakeSet
      en:VACC_ACCSetTimeGap_enum=TimeGapPosn;
      en:VACC_ACCSetTimeGapTmp_enum=VACC_ACCSetTimeGap_enum;
    state DistanceSet
      state WaitingForTimeGapChange
        en:VACC_ACCSetTimeGap_enum=VACC_ACCSetTimeGapTmp_enum;
      state PrepareToDec
      state Decrease1
        en: TimeGapPosn=TimeGapPosn-1;
      state Increase
        en: TimeGapPosn=TimeGapPosn+1;
      state SignChangePlus
        en:TimeGapPosn=1;
        en:VACC_ACCSetTimeGapSignIni_flg=TRUE;
      state SignChangeMinus
        en:TimeGapPosn=4;
        en:VACC_ACCSetTimeGapSignIni_flg=FALSE;
      state WaitingForTimeGapChangeTmp
        en:VACC_ACCSetTimeGapTmp_enum=TimeGapPosn;
      (default) -> WaitingForTimeGapChange
      (junction 261) -> WaitingForTimeGapChange [order 1] : after(VACC_TimeGapChgTimeThres_s/C_TASK_5MS_S,tick) ...
          | [!VACC_ACCTimeGapDecVCU_flg]
      WaitingForTimeGapChange -> (junction 262) : [VACC_ACCTimeGapDecVCU_flg]
      (junction 261) -> (junction 262) [order 2] : [VACC_ACCTimeGapDecVCU_flg]
      WaitingForTimeGapChangeTmp -> (junction 261)
      (junction 262) -> PrepareToDec
      PrepareToDec -> (junction 263) : [!VACC_ACCTimeGapDecVCU_flg]
      (junction 263) -> (junction 264) [order 1] : [VACC_ACCSetTimeGapSignLast_flg==TRUE]
      (junction 264) -> SignChangeMinus [order 2]
      (junction 263) -> (junction 265) [order 2] : [VACC_ACCSetTimeGapSignLast_flg==FALSE]
      (junction 264) -> Increase [order 1] : [TimeGapPosn<4]
      (junction 265) -> SignChangePlus [order 2]
      (junction 265) -> Decrease1 [order 1] : [TimeGapPosn>1]
      Decrease1 -> (junction 266)
      Increase -> (junction 267)
      (junction 266) -> WaitingForTimeGapChangeTmp [order 2]
      (junction 267) -> WaitingForTimeGapChangeTmp [order 2]
      (junction 266) -> SignChangePlus [order 1] : [TimeGapPosn==1]
      (junction 267) -> SignChangeMinus [order 1] : [TimeGapPosn==4]
      SignChangeMinus -> WaitingForTimeGapChangeTmp
      SignChangePlus -> WaitingForTimeGapChangeTmp
    (default) -> WaitforACCActive
    (junction 241) -> WaitforACCActive
    (junction 246) -> (junction 241)
    WaitforACCActive -> (junction 242)
    (junction 242) -> (junction 243) [order 1] : [(VACC_ACCTimeGapIncVCU_flg || VACC_ACCTimeGapDecVCU_flg) && VDINR_DriverBrakPedalOn_flg && VACC_InPNGear_flg && (VDINR_VehSpd_kph<VACC_SetAllowSpdLim_kph)]
    (junction 242) -> (junction 244) [order 2] : [VACC_ACCActivated_flg]
    (junction 243) -> BrakeSet
    (junction 244) -> (junction 245) [order 1] : [VACC_ACCResOn_flg]
    (junction 244) -> SetOn [order 2] : [!VACC_ACCResOn_flg]
    (junction 245) -> ResOn
    SetOn -> DistanceSet : [!VACC_ACCTimeGapIncVCU_flg &&...
        | !VACC_ACCTimeGapDecVCU_flg]
    ResOn -> DistanceSet : [!VACC_ACCTimeGapIncVCU_flg &&...
        | !VACC_ACCTimeGapDecVCU_flg]
    BrakeSet -> DistanceSet : [!VACC_ACCTimeGapIncVCU_flg &&...
        | !VACC_ACCTimeGapDecVCU_flg]
    DistanceSet -> (junction 246) : [!VACC_ACCActivated_flg && ...
        | (!VDINR_DriverBrakPedalOn_flg || ...
        | VDINR_VehSpd_kph>=VACC_SetAllowSpdLim_kph ||...
        | !VACC_InPNGear_flg)]
  (default) -> Initialize
  Initialize -> ACCOn : [VACC_ACCStatus_enum==ENUM_ACCSTATUS_STANDBY || ...
      | VACC_ACCStatus_enum==ENUM_ACCSTATUS_ACTIVE]
  ACCOff -> ACCOn : [VACC_ACCStatus_enum==ENUM_ACCSTATUS_STANDBY || ...
      | VACC_ACCStatus_enum==ENUM_ACCSTATUS_ACTIVE]
  ACCOn -> ACCOff : [VACC_ACCStatus_enum==ENUM_ACCSTATUS_OFF]
  data: VACC_ACCStatus_enum input double; VACC_ACCActivated_flg input double; VACC_ACCResOn_flg input double; VDINR_DriverBrakPedalOn_flg input double; VDINR_VehSpd_kph input double; VACC_InPNGear_flg input double; VACC_ACCSetTimeGap_enum output double; VACC_ACCTimeGapIncVCU_flg input double; VACC_ACCTimeGapDecVCU_flg input double; TimeGapPosn local uint8; VACC_ACCSetTimeGapTmp_enum output double; VACC_ACCSetTimeGapSignIni_flg output boolean; C_TASK_5MS_S parameter double; VACC_TimeGapChgTimeThres_s input double; VACC_SetAllowSpdLim_kph input double; VACC_ACCSetTimeGapSignLast_flg input double; ENUM_ACCSTATUS_STANDBY parameter double; ENUM_ACCSTATUS_ACTIVE parameter double; ENUM_ACCSTATUS_OFF parameter double; TRUE parameter double; FALSE parameter double

== stateflow chart EPSS/EPSS/AngleMode/Angle2Torque/Rate_Limit/RateLimiter/Chart ==
  state Increase
    en:
    tou=increase_tou;
    Max=Data_in;
    Min=-10000000000;
    Initial=0;
    du:
    tou=increase_tou;
    Max=Data_in;
    Min=-10000000000;
    Initial=0;
  state Decrease
    en:
    tou=decrease_tou;
    Max=10000000000;
    Min=Data_in;
    Initial=0;
    du:
    tou=decrease_tou;
    Max=10000000000;
    Min=Data_in;
    Initial=0;
  state Start
    en:
    tou=0;
    Max=10000000000;
    Min=-10000000000;
    Initial=1;
  (default) -> Start
  Start -> Increase [order 2] : [increase]
  Start -> Decrease [order 1] : [decrease]
  Increase -> Decrease : [decrease]
  Decrease -> Increase : [increase]
  data: Initial output double; increase input double; decrease input double; Data_in input double; increase_tou input double; decrease_tou input double; tou output double; Min output double; Max output double

== stateflow chart APPH/ACC/ACC/ACCStatus_SetSpeed_SetTimeGap/ACC_State_Determination ==
  state ACCStandBy
    state WaitForSet
      en:VACC_ACCStatus_enum=ENUM_ACCSTATUS_STANDBY;
      en:VACC_ACCActivated_flg=FALSE;
      en:VACC_ACCResOn_flg=FALSE;
    state ACCSet
      en:VACC_ACCStatus_enum=ENUM_ACCSTATUS_ACTIVE;
      en:VACC_ACCActivated_flg=TRUE;
      en:VACC_ACCResOn_flg=FALSE;
    state ACCRes
      en:VACC_ACCStatus_enum=ENUM_ACCSTATUS_ACTIVE;
      en:VACC_ACCActivated_flg=TRUE;
      en:VACC_ACCResOn_flg=TRUE;
    (default) -> WaitForSet
    WaitForSet -> ACCSet [order 1] : [VACC_ACCSetSpdDecVCU_flg && ...
        | !VDINR_DriverBrakPedalOn_flg && ...
        | !VAEB_AEBActive_flg && ...
        | VACC_InForwardGear_flg && ...
        | VDINR_VehSpd_kph>=VACC_MinAccSetSpd_kph && ...
        | VDINR_VehSpd_kph<=VACC_MaxAccSetSpd_kph]
    ACCSet -> WaitForSet : [VDINR_DriverBrakPedalOn_flg || ...
        | VAEB_AEBActive_flg || ...
        | !VACC_InForwardGear_flg]
    WaitForSet -> ACCRes [order 2] : [VACC_ACCResSpdIncVCU_flg && ...
        | !VDINR_DriverBrakPedalOn_flg && ...
        | !VAEB_AEBActive_flg && ...
        | VACC_InForwardGear_flg && ...
        | VDINR_VehSpd_kph<=VACC_MaxAccSetSpd_kph && ...
        | VACC_ACCSetSpd_kph~=0 && ...
        | VACC_ACCSetTimeGap_enum~=0]
    ACCRes -> WaitForSet : [VDINR_DriverBrakPedalOn_flg || ...
        | VAEB_AEBActive_flg || ...
        | !VACC_InForwardGear_flg]
  state ACCOff
    en:VACC_ACCStatus_enum=ENUM_ACCSTATUS_OFF;
    en:VACC_ACCActivated_flg=FALSE;
    en:VACC_ACCResOn_flg=FALSE;
  (default) -> ACCOff
  ACCOff -> ACCStandBy : [VACC_ACCOnVCU_flg]
  ACCStandBy -> ACCOff : [!VACC_ACCOnVCU_flg]
  data: VACC_ACCStatus_enum output double; VDINR_DriverBrakPedalOn_flg input double; VAEB_AEBActive_flg input double; VACC_InForwardGear_flg input double; VACC_ACCActivated_flg output double; VACC_ACCOnVCU_flg input double; VDINR_VehSpd_kph input double; VACC_ACCSetSpdDecVCU_flg input double; VACC_ACCResSpdIncVCU_flg input double; VACC_ACCResOn_flg output double; TRUE parameter double; FALSE parameter double; ENUM_ACCSTATUS_OFF parameter double; ENUM_ACCSTATUS_STANDBY parameter double; ENUM_ACCSTATUS_ACTIVE parameter double; VACC_ACCSetSpd_kph input double; VACC_ACCSetTimeGap_enum input double; VACC_MinAccSetSpd_kph input double; VACC_MaxAccSetSpd_kph input double

== stateflow chart APPH/ACC/ACC/ACCStatus_SetSpeed_SetTimeGap/ACCOnSwitchLatch ==
  state WaitingOn
    en:VACC_ACCOnVCU_flg=FALSE;
  state ACCOn
    en:VACC_ACCOnVCU_flg=TRUE;
  state WaitingOff
    en:VACC_ACCOnVCU_flg=TRUE;
  state ACCOff
    en:VACC_ACCOnVCU_flg=FALSE;
  (default) -> WaitingOn
  WaitingOn -> ACCOn : [VDINR_ACCOnVCU_flg]
  ACCOn -> WaitingOff : [!VDINR_ACCOnVCU_flg]
  (junction 377) -> WaitingOn
  WaitingOff -> (junction 378)
  ACCOff -> (junction 377) : [!VDINR_ACCOnVCU_flg]
  (junction 378) -> ACCOff : [VDINR_ACCOnVCU_flg]
  data: VACC_ACCOnVCU_flg output double; VDINR_ACCOnVCU_flg input double; TRUE parameter double; FALSE parameter double

== stateflow chart APPH/ACC/ACC/ACCStatus_SetSpeed_SetTimeGap/ACC_SetTimeGap_Determination ==
  (default) -> (junction 395)
  (junction 395) -> (junction 396) [order 1] : [VACC_ACCSetTimeGap_enum==0]
  (junction 395) -> (junction 397) [order 2]
  (junction 396) -> (junction 410) : {VACC_ACCSetTimeGap_s= ...
      | single(999);}
  (junction 397) -> (junction 398) [order 1] : [VACC_ACCSetTimeGap_enum==1]
  (junction 397) -> (junction 399) [order 2]
  (junction 398) -> (junction 409) : {VACC_ACCSetTimeGap_s= ...
      | VACC_ACCSetTimeGapDef1_s;}
  (junction 399) -> (junction 400) [order 1] : [VACC_ACCSetTimeGap_enum==2]
  (junction 399) -> (junction 401) [order 2]
  (junction 400) -> (junction 408) : {VACC_ACCSetTimeGap_s= ...
      | VACC_ACCSetTimeGapDef2_s;}
  (junction 401) -> (junction 402) [order 1] : [VACC_ACCSetTimeGap_enum==3]
  (junction 401) -> (junction 403) [order 2]
  (junction 402) -> (junction 407) : {VACC_ACCSetTimeGap_s= ...
      | VACC_ACCSetTimeGapDef3_s;}
  (junction 403) -> (junction 404) [order 1] : [VACC_ACCSetTimeGap_enum==4]
  (junction 403) -> (junction 405) [order 2] : {VACC_ACCSetTimeGap_s= ...
      | VACC_ACCSetTimeGapDef5_s;}
  (junction 404) -> (junction 406) : {VACC_ACCSetTimeGap_s= ...
      | VACC_ACCSetTimeGapDef4_s;}
  (junction 406) -> (junction 405)
  (junction 407) -> (junction 406)
  (junction 408) -> (junction 407)
  (junction 409) -> (junction 408)
  (junction 410) -> (junction 409)
  data: VACC_ACCSetTimeGap_enum input double; VACC_ACCSetTimeGapDef1_s input double; VACC_ACCSetTimeGapDef2_s input double; VACC_ACCSetTimeGapDef3_s input double; VACC_ACCSetTimeGapDef4_s input double; VACC_ACCSetTimeGapDef5_s input double; VACC_ACCSetTimeGap_s output double
